simulink model "ESSController"  (R2020a)
settings: Solver=FixedStepAuto  StartTime=0.0  StopTime=10.0  FixedStep=1  RelTol=1e-3
libraries: ESSLibrary x19, simulink x1
settings Model: DataDictionary=ESSControllerData.sldd  EnableAccessToBaseWorkspace=off  Creator=soumyakantapanda  LastModifiedBy=soumyakantapanda

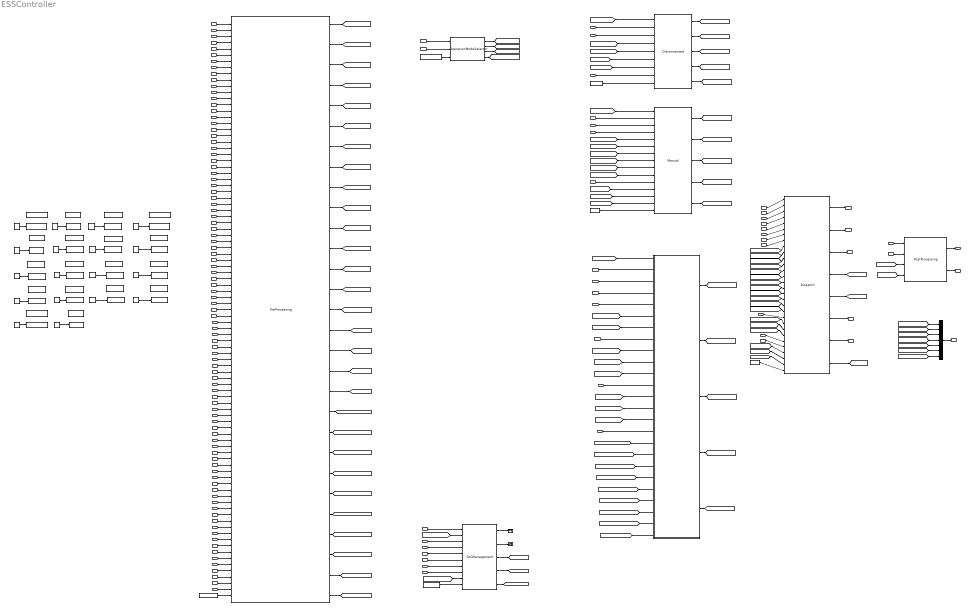
== system ESSController ==
  note: Dispatch and PostProcessing
  note: Auto Mode
  note: Manual Mode
  note: Disconnected Mode
  note: State of Charge Management Block
  note: Operation Mode Selection
  note: Pre-Processing
  note: LogicBlockIDGenerator
  EnablePreProcessing : Inport
  ActivePowerSet : Inport  Port=2
  ReactivePowerSet : Inport  Port=3
  ActivePowerMeasECP : Inport  Port=4
  ReactivePowerMeasECP : Inport  Port=5
  ActivePowerMeasCtrlPoint : Inport  Port=6
  ReactivePowerMeasCtrlPoint : Inport  Port=7
  FreqMeas : Inport  Port=8
  VoltMeasECPL1 : Inport  Port=9
  VoltMeasECPL2 : Inport  Port=10
  VoltMeasECPL3 : Inport  Port=11
  MaxDischargingPower : Inport  Port=12
  MaxChargingPower : Inport  Port=13
  ECPAppPow : Inport  Port=14
  RefFreq : Inport  Port=15
  RefVolt : Inport  Port=16
  TimeStep : Inport  Port=17
  BreakerCmdTime : Inport  Port=18
  OpenTimeOut : Inport  Port=19
  CloseTimeOut : Inport  Port=20
  ActivePowerRampUpRate : Inport  Port=21
  ActivePowerRampDownRate : Inport  Port=22
  ReactivePowerRampUpRate : Inport  Port=23
  ReactivePowerRampDownRate : Inport  Port=24
  VoltCloseThreshold : Inport  Port=25
  FreqCloseThreshold : Inport  Port=26
  ActivePowerOpenThreshold : Inport  Port=27
  ReactivePowerOpenThreshold : Inport  Port=28
  PQCapabilityCurveP1 : Inport  Port=29
  PQCapabilityCurveQ1 : Inport  Port=30
  PQCapabilityCurveP2 : Inport  Port=31
  PQCapabilityCurveQ2 : Inport  Port=32
  PQCapabilityCurveP3 : Inport  Port=33
  PQCapabilityCurveQ3 : Inport  Port=34
  PQCapabilityCurveP4 : Inport  Port=35
  PQCapabilityCurveQ4 : Inport  Port=36
  PQCapabilityCurveP5 : Inport  Port=37
  PQCapabilityCurveQ5 : Inport  Port=38
  PQCapabilityCurveP6 : Inport  Port=39
  PQCapabilityCurveQ6 : Inport  Port=40
  PQCapabilityCurveP7 : Inport  Port=41
  PQCapabilityCurveQ7 : Inport  Port=42
  PQCapabilityCurveP8 : Inport  Port=43
  PQCapabilityCurveQ8 : Inport  Port=44
  SoCTarget : Inport  Port=45
  MaxChOrDischDuration : Inport  Port=46
  BattCapacity : Inport  Port=47
  MaxImportPower : Inport  Port=48
  MaxExportPower : Inport  Port=49
  ActivePowerResponseReductionRatio : Inport  Port=50
  ActivePowerSmoothingLowDeadBand : Inport  Port=51
  ActivePowerSmoothingHighDeadBand : Inport  Port=52
  ActivePowerSmoothingGradient : Inport  Port=53
  ActivePowerSmoothingMovingAverageWindow : Inport  Port=54
  VoltWattHiStartVoltage : Inport  Port=55
  VoltWattHiStopVoltage : Inport  Port=56
  VoltWattHiVoltDischargeGradient : Inport  Port=57
  VoltWattHiVoltChargeGradient : Inport  Port=58
  VoltWattLoStartVoltage : Inport  Port=59
  VoltWattLoStopVoltage : Inport  Port=60
  VoltWattLoVoltDischargeGradient : Inport  Port=61
  VoltWattLoVoltChargeGradient : Inport  Port=62
  VoltWattStartDelay : Inport  Port=63
  VoltWattStopDelay : Inport  Port=64
  FreqWattHiStartFreq : Inport  Port=65
  FreqWattHiStopFreq : Inport  Port=66
  FreqWattHiFreqDischargeGradient : Inport  Port=67
  FreqWattHiFreqChargeGradient : Inport  Port=68
  FreqWattLoStartFreq : Inport  Port=69
  FreqWattLoStopFreq : Inport  Port=70
  FreqWattLoFreqDischargeGradient : Inport  Port=71
  FreqWattLoFreqChargeGradient : Inport  Port=72
  FreqWattStartDelay : Inport  Port=73
  FreqWattStopDelay : Inport  Port=74
  DynamicVoltWattLowDeadBand : Inport  Port=75
  DynamicVoltWattHighDeadBand : Inport  Port=76
  DynamicVoltWattGradient : Inport  Port=77
  DynamicVoltWattMovingAverageWindow : Inport  Port=78
  VoltVarHighStartingVoltage : Inport  Port=79
  VoltVarHighStoppingVoltage : Inport  Port=80
  VoltVarHighVoltageGradient : Inport  Port=81
  VoltVarLowStartingVoltage : Inport  Port=82
  VoltVarLowStoppingVoltage : Inport  Port=83
  VoltVarLowVoltageGradient : Inport  Port=84
  VoltVarOffsetReactivePower : Inport  Port=85
  WattVarHighStartingWattage : Inport  Port=86
  WattVarHighStoppingWattage : Inport  Port=87
  WattVarHighWattageGradient : Inport  Port=88
  WattVarLowStartingWattage : Inport  Port=89
  WattVarLowStoppingWattage : Inport  Port=90
  WattVarLowWattgeGradient : Inport  Port=91
  WattVarOffsetReactivePower : Inport  Port=92
  EnableOperationModeSelector : Inport  Port=93
  OperationMode : Inport  Port=94
  EnableSoCManagement : Inport  Port=95
  SoCMeas : Inport  Port=96
  SoCMin : Inport  Port=97
  SoCMax : Inport  Port=98
  CommQual : Inport  Port=99
  CBStatus : Inport  Port=100
  ResetDisconnected : Inport  Port=101
  OpenCmdIn : Inport  Port=102
  CloseCmdIn : Inport  Port=103
  ActivePowerControlMode : Inport  Port=104
  ReactivePowerControlMode : Inport  Port=105
  PowerFactorSet : Inport  Port=106
  ActivePowerLimitChargeOrDischarge : Inport  Port=107
  EnableDispatch : Inport  Port=108
  EnableRampLimiter : Inport  Port=109
  EnablePQCapabilityCurve : Inport  Port=110
  PQPriority : Inport  Port=111
  EnablePFLimit : Inport  Port=112
  PFOperMax : Inport  Port=113
  PFOperMin : Inport  Port=114
  EnablePostProcessing : Inport  Port=115
  ActivePowerControlMode1 : InportShadow  Port=104
  Auto : Subsystem
  BattCapacity1 : InportShadow  Port=47
  CBStatus1 : InportShadow  Port=100
  CBStatus2 : InportShadow  Port=100
  CommQual1 : InportShadow  Port=99
  CommQual2 : InportShadow  Port=99
  CommQual3 : InportShadow  Port=99
  Constant2 : Constant  OutDataTypeStr=int32  SampleTime=-1
  Constant3 : Constant  Value=2  OutDataTypeStr=int32  SampleTime=-1
  Constant37 : Constant  Value=7  OutDataTypeStr=int32  SampleTime=-1
  Constant38 : Constant  Value=8  OutDataTypeStr=int32  SampleTime=-1
  Constant4 : Constant  Value=3  OutDataTypeStr=int32  SampleTime=-1
  Constant40 : Constant  Value=9  OutDataTypeStr=int32  SampleTime=-1
  Constant41 : Constant  Value=10  OutDataTypeStr=int32  SampleTime=-1
  Constant42 : Constant  Value=11  OutDataTypeStr=int32  SampleTime=-1
  Constant43 : Constant  Value=12  OutDataTypeStr=int32  SampleTime=-1
  Constant44 : Constant  Value=13  OutDataTypeStr=int32  SampleTime=-1
  Constant45 : Constant  Value=14  OutDataTypeStr=int32  SampleTime=-1
  Constant46 : Constant  Value=15  OutDataTypeStr=int32  SampleTime=-1
  Constant47 : Constant  Value=16  OutDataTypeStr=int32  SampleTime=-1
  Constant48 : Constant  Value=17  OutDataTypeStr=int32  SampleTime=-1
  Constant5 : Constant  Value=4  OutDataTypeStr=int32  SampleTime=-1
  Constant6 : Constant  Value=5  OutDataTypeStr=int32  SampleTime=-1
  Constant8 : Constant  Value=18  OutDataTypeStr=int32  SampleTime=-1
  Constant9 : Constant  Value=8  OutDataTypeStr=int64  SampleTime=-1
  Data Store Memory2 : DataStoreMemory  DataStoreName=OperationModeSelector  ShowAdditionalParam=off
  Data Store Memory3 : DataStoreMemory  DataStoreName=SoCComparator  ShowAdditionalParam=off
  Data Store Memory35 : DataStoreMemory  DataStoreName=ChargeDischargeStorageMode  ShowAdditionalParam=off
  Data Store Memory36 : DataStoreMemory  DataStoreName=CoordinatedChDisMode  ShowAdditionalParam=off
  Data Store Memory38 : DataStoreMemory  DataStoreName=ActivePowResponseMode  ShowAdditionalParam=off
  Data Store Memory39 : DataStoreMemory  DataStoreName=ActivePowSmoothingMode  ShowAdditionalParam=off
  Data Store Memory4 : DataStoreMemory  DataStoreName=PreProcessingBlock  ShowAdditionalParam=off
  Data Store Memory40 : DataStoreMemory  DataStoreName=VoltWattMode  ShowAdditionalParam=off
  Data Store Memory41 : DataStoreMemory  DataStoreName=FreqWattMode  ShowAdditionalParam=off
  Data Store Memory42 : DataStoreMemory  DataStoreName=DynamicVoltWattMode  ShowAdditionalParam=off
  Data Store Memory43 : DataStoreMemory  DataStoreName=ConstVARMode  ShowAdditionalParam=off
  Data Store Memory44 : DataStoreMemory  DataStoreName=FixedPFMode  ShowAdditionalParam=off
  Data Store Memory45 : DataStoreMemory  DataStoreName=VoltVARMode  ShowAdditionalParam=off
  Data Store Memory46 : DataStoreMemory  DataStoreName=WattVARMode  ShowAdditionalParam=off
  Data Store Memory5 : DataStoreMemory  DataStoreName=Disconnected  ShowAdditionalParam=off
  Data Store Memory6 : DataStoreMemory  DataStoreName=Manual  ShowAdditionalParam=off
  Data Store Memory8 : DataStoreMemory  DataStoreName=Dispatch  ShowAdditionalParam=off
  Data Store Memory9 : DataStoreMemory  DataStoreName=PostProcessing  ShowAdditionalParam=off
  Data Store Read : DataStoreRead  DataStoreName=PreProcessingBlock
  Data Store Read1 : DataStoreRead  DataStoreName=OperationModeSelector
  Data Store Read2 : DataStoreRead  DataStoreName=SoCComparator
  Data Store Read3 : DataStoreRead  DataStoreName=Disconnected
  Data Store Read4 : DataStoreRead  DataStoreName=Manual
  Data Store Read5 : DataStoreRead  DataStoreName=Dispatch
  Data Store Write2 : DataStoreWrite  DataStoreName=SoCComparator
  Data Store Write3 : DataStoreWrite  DataStoreName=OperationModeSelector
  Data Store Write35 : DataStoreWrite  DataStoreName=ChargeDischargeStorageMode
  Data Store Write36 : DataStoreWrite  DataStoreName=CoordinatedChDisMode
  Data Store Write38 : DataStoreWrite  DataStoreName=ActivePowResponseMode
  Data Store Write39 : DataStoreWrite  DataStoreName=ActivePowSmoothingMode
  Data Store Write4 : DataStoreWrite  DataStoreName=PreProcessingBlock
  Data Store Write40 : DataStoreWrite  DataStoreName=VoltWattMode
  Data Store Write41 : DataStoreWrite  DataStoreName=FreqWattMode
  Data Store Write42 : DataStoreWrite  DataStoreName=DynamicVoltWattMode
  Data Store Write43 : DataStoreWrite  DataStoreName=ConstVARMode
  Data Store Write44 : DataStoreWrite  DataStoreName=FixedPFMode
  Data Store Write45 : DataStoreWrite  DataStoreName=VoltVARMode
  Data Store Write46 : DataStoreWrite  DataStoreName=WattVARMode
  Data Store Write5 : DataStoreWrite  DataStoreName=Manual
  Data Store Write6 : DataStoreWrite  DataStoreName=Disconnected
  Data Store Write8 : DataStoreWrite  DataStoreName=PostProcessing
  Data Store Write9 : DataStoreWrite  DataStoreName=Dispatch
  Disconnected : ESSLibrary/Disconnected  SystemSampleTime=-1  Latency=0  AutoFrameSizeCalculation=off
  Dispatch : ESSLibrary/Dispatch  SystemSampleTime=-1  Latency=0  AutoFrameSizeCalculation=off
  ECPAppPow1 : InportShadow  Port=14
  ECPAppPow2 : InportShadow  Port=14
  Manual : ESSLibrary/Manual  SystemSampleTime=-1  Latency=0  AutoFrameSizeCalculation=off
  Mux : Mux  Inputs=7
  OperationMode1 : InportShadow  Port=94
  OperationModeSelector : ESSLibrary/OperationModeSelector  SystemSampleTime=-1  Latency=0  AutoFrameSizeCalculation=off
  PostProcessing : ESSLibrary/PostProcessing  SystemSampleTime=-1  Latency=0  AutoFrameSizeCalculation=off
  PreProcessing : ESSLibrary/PreProcessing  SystemSampleTime=-1  Latency=0  AutoFrameSizeCalculation=off
  ReactivePowerControlMode1 : InportShadow  Port=105
  SoCManagement : ESSLibrary/SoCManagement  SystemSampleTime=-1  Latency=0  AutoFrameSizeCalculation=off
  SoCMeas1 : InportShadow  Port=96
  Terminator : Terminator
  Terminator1 : Terminator
  TimeStep1 : InportShadow  Port=17
  OperationModeOut : Outport  SignalName=OperationModeOut
  ActivePowerModeOut : Outport  Port=2  SignalName=ActivePowerModeOut
  ReactivePowerModeOut : Outport  Port=3  SignalName=ReactivePowerModeOut
  OpenCmdOut : Outport  Port=4  SignalName=OpenCmdOut
  CloseCmdOut : Outport  Port=5  SignalName=CloseCmdOut
  ActivePowerOut : Outport  Port=6  SignalName=ActivePowerOut
  ReactivePowerOut : Outport  Port=7  SignalName=ReactivePowerOut
  ErrorCode : Outport  Port=8  SignalName=ErrorCode
  wires:
  Constant38/1 -> Data Store Write36/1
  Constant8/1 -> Data Store Write9/1
  Constant43/1 -> Data Store Write41/1
  Constant42/1 -> Data Store Write40/1
  Constant48/1 -> Data Store Write46/1
  Constant47/1 -> Data Store Write45/1
  Constant46/1 -> Data Store Write44/1
  Constant45/1 -> Data Store Write43/1
  Constant40/1 -> Data Store Write38/1
  Constant44/1 -> Data Store Write42/1
  Constant37/1 -> Data Store Write35/1
  Constant2/1 -> Data Store Write3/1
  Constant6/1 -> Data Store Write5/1
  Constant3/1 -> Data Store Write2/1
  Constant5/1 -> Data Store Write6/1
  Constant9/1 -> Data Store Write8/1
  Constant41/1 -> Data Store Write39/1
  Constant4/1 -> Data Store Write4/1
  EnablePreProcessing/1 -> PreProcessing/1
  ActivePowerSet/1 -> PreProcessing/2
  ReactivePowerSet/1 -> PreProcessing/3
  ActivePowerMeasECP/1 -> PreProcessing/4
  ReactivePowerMeasECP/1 -> PreProcessing/5
  ActivePowerMeasCtrlPoint/1 -> PreProcessing/6
  ReactivePowerMeasCtrlPoint/1 -> PreProcessing/7
  FreqMeas/1 -> PreProcessing/8
  VoltMeasECPL1/1 -> PreProcessing/9
  VoltMeasECPL2/1 -> PreProcessing/10
  VoltMeasECPL3/1 -> PreProcessing/11
  MaxDischargingPower/1 -> PreProcessing/12
  ReactivePowerRampDownRate/1 -> PreProcessing/24
  ReactivePowerRampUpRate/1 -> PreProcessing/23
  ActivePowerRampDownRate/1 -> PreProcessing/22
  ActivePowerRampUpRate/1 -> PreProcessing/21
  CloseTimeOut/1 -> PreProcessing/20
  OpenTimeOut/1 -> PreProcessing/19
  BreakerCmdTime/1 -> PreProcessing/18
  TimeStep/1 -> PreProcessing/17
  RefVolt/1 -> PreProcessing/16
  RefFreq/1 -> PreProcessing/15
  ECPAppPow/1 -> PreProcessing/14
  MaxChargingPower/1 -> PreProcessing/13
  PQCapabilityCurveP5/1 -> PreProcessing/37
  PQCapabilityCurveQ5/1 -> PreProcessing/38
  PQCapabilityCurveP6/1 -> PreProcessing/39
  PQCapabilityCurveQ6/1 -> PreProcessing/40
  PQCapabilityCurveP7/1 -> PreProcessing/41
  PQCapabilityCurveQ7/1 -> PreProcessing/42
  PQCapabilityCurveP8/1 -> PreProcessing/43
  PQCapabilityCurveQ8/1 -> PreProcessing/44
  SoCTarget/1 -> PreProcessing/45
  MaxChOrDischDuration/1 -> PreProcessing/46
  BattCapacity/1 -> PreProcessing/47
  MaxImportPower/1 -> PreProcessing/48
  PQCapabilityCurveQ4/1 -> PreProcessing/36
  PQCapabilityCurveP4/1 -> PreProcessing/35
  PQCapabilityCurveQ3/1 -> PreProcessing/34
  PQCapabilityCurveP3/1 -> PreProcessing/33
  PQCapabilityCurveQ2/1 -> PreProcessing/32
  PQCapabilityCurveP2/1 -> PreProcessing/31
  PQCapabilityCurveQ1/1 -> PreProcessing/30
  PQCapabilityCurveP1/1 -> PreProcessing/29
  ReactivePowerOpenThreshold/1 -> PreProcessing/28
  ActivePowerOpenThreshold/1 -> PreProcessing/27
  FreqCloseThreshold/1 -> PreProcessing/26
  VoltCloseThreshold/1 -> PreProcessing/25
  FreqWattStartDelay/1 -> PreProcessing/73
  FreqWattStopDelay/1 -> PreProcessing/74
  DynamicVoltWattLowDeadBand/1 -> PreProcessing/75
  DynamicVoltWattHighDeadBand/1 -> PreProcessing/76
  DynamicVoltWattGradient/1 -> PreProcessing/77
  DynamicVoltWattMovingAverageWindow/1 -> PreProcessing/78
  VoltVarHighStartingVoltage/1 -> PreProcessing/79
  VoltVarHighStoppingVoltage/1 -> PreProcessing/80
  VoltVarHighVoltageGradient/1 -> PreProcessing/81
  VoltVarLowStartingVoltage/1 -> PreProcessing/82
  VoltVarLowStoppingVoltage/1 -> PreProcessing/83
  VoltVarLowVoltageGradient/1 -> PreProcessing/84
  Data Store Read/1 -> PreProcessing/93
  WattVarOffsetReactivePower/1 -> PreProcessing/92
  WattVarLowWattgeGradient/1 -> PreProcessing/91
  WattVarLowStoppingWattage/1 -> PreProcessing/90
  WattVarLowStartingWattage/1 -> PreProcessing/89
  WattVarHighWattageGradient/1 -> PreProcessing/88
  WattVarHighStoppingWattage/1 -> PreProcessing/87
  WattVarHighStartingWattage/1 -> PreProcessing/86
  VoltVarOffsetReactivePower/1 -> PreProcessing/85
  VoltWattLoVoltDischargeGradient/1 -> PreProcessing/61
  VoltWattLoVoltChargeGradient/1 -> PreProcessing/62
  VoltWattStartDelay/1 -> PreProcessing/63
  VoltWattStopDelay/1 -> PreProcessing/64
  FreqWattHiStartFreq/1 -> PreProcessing/65
  FreqWattHiStopFreq/1 -> PreProcessing/66
  FreqWattHiFreqDischargeGradient/1 -> PreProcessing/67
  FreqWattHiFreqChargeGradient/1 -> PreProcessing/68
  FreqWattLoStartFreq/1 -> PreProcessing/69
  FreqWattLoStopFreq/1 -> PreProcessing/70
  FreqWattLoFreqDischargeGradient/1 -> PreProcessing/71
  FreqWattLoFreqChargeGradient/1 -> PreProcessing/72
  VoltWattLoStopVoltage/1 -> PreProcessing/60
  VoltWattLoStartVoltage/1 -> PreProcessing/59
  VoltWattHiVoltChargeGradient/1 -> PreProcessing/58
  VoltWattHiVoltDischargeGradient/1 -> PreProcessing/57
  VoltWattHiStopVoltage/1 -> PreProcessing/56
  VoltWattHiStartVoltage/1 -> PreProcessing/55
  ActivePowerSmoothingMovingAverageWindow/1 -> PreProcessing/54
  ActivePowerSmoothingGradient/1 -> PreProcessing/53
  ActivePowerSmoothingHighDeadBand/1 -> PreProcessing/52
  ActivePowerSmoothingLowDeadBand/1 -> PreProcessing/51
  ActivePowerResponseReductionRatio/1 -> PreProcessing/50
  MaxExportPower/1 -> PreProcessing/49
  PreProcessing/1 -> [ActivePowerSetPU]
  PreProcessing/2 -> [ReactivePowerSetPU]
  PreProcessing/3 -> [ActivePowerMeasPU]
  PreProcessing/4 -> [ReactivePowerMeasPU]
  PreProcessing/5 -> [ActivePowerMeasCtrlPointPU]
  PreProcessing/6 -> [ReactivePowerMeasCtrlPointPU]
  PreProcessing/7 -> [FreqMeasPU]
  PreProcessing/8 -> [VoltMeasPU]
  PreProcessing/9 -> [MaxDischargingPowerPU]
  PreProcessing/10 -> [MaxChargingPowerPU]
  PreProcessing/11 -> [FreqWithinLimits]
  PreProcessing/12 -> [VoltWithinLimits]
  PreProcessing/13 -> [ZeroActivePowerFlow]
  PreProcessing/14 -> [ZeroReactivePowerFlow]
  PreProcessing/15 -> [ActiveReactiveRampUpDownData]
  PreProcessing/16 -> [PQCapabilityCurvePU]
  PreProcessing/17 -> [BreakerCmdTimeSteps]
  PreProcessing/18 -> [OpenTimeOutTimeSteps]
  PreProcessing/19 -> [CloseTimeOutTimeSteps]
  PreProcessing/20 -> [ActivePowerLimitOperatingParametersPU]
  PreProcessing/21 -> [CrdChargeDischargeOperatingParametersPU]
  PreProcessing/22 -> [ActivePowerResponseOperatingParametersPU]
  PreProcessing/23 -> [ActivePowerSmoothingOperatingParametersPU]
  PreProcessing/24 -> [VoltWattOperatingParametersPU]
  PreProcessing/25 -> [FreqWattOperatingParametersPU]
  PreProcessing/26 -> [DynamicVoltWattOperatingParametersPU]
  PreProcessing/27 -> [VoltVAROperatingParametersPU]
  PreProcessing/28 -> [WattVAROperatingParametersPU]
  PreProcessing/29 -> [PreProcessingErrorCode]
  EnableOperationModeSelector/1 -> OperationModeSelector/1
  OperationMode/1 -> OperationModeSelector/2
  Data Store Read1/1 -> OperationModeSelector/3
  OperationModeSelector/3 -> [EnableAutoMode]
  OperationModeSelector/1 -> [EnableDisconnectedMode]
  OperationModeSelector/4 -> [OperationModeSelectorErrorCode]
  OperationModeSelector/2 -> [EnableManualMode]
  EnableSoCManagement/1 -> SoCManagement/1
  [ActivePowerMeasPU] -> SoCManagement/2
  SoCMeas/1 -> SoCManagement/3
  SoCMin/1 -> SoCManagement/4
  SoCMax/1 -> SoCManagement/5
  BattCapacity1/1 -> SoCManagement/6
  ECPAppPow1/1 -> SoCManagement/7
  TimeStep1/1 -> SoCManagement/8
  [ActiveReactiveRampUpDownData] -> SoCManagement/9
  Data Store Read2/1 -> SoCManagement/10
  SoCManagement/1 -> Terminator/1
  SoCManagement/2 -> Terminator1/1
  SoCManagement/3 -> [ChargeEnable]
  SoCManagement/4 -> [DischargeEnable]
  SoCManagement/5 -> [SoCManagementErrorCode]
  [EnableDisconnectedMode] -> Disconnected/1
  CommQual/1 -> Disconnected/2
  CBStatus/1 -> Disconnected/3
  [ZeroActivePowerFlow] -> Disconnected/4
  [ZeroReactivePowerFlow] -> Disconnected/5
  [BreakerCmdTimeSteps] -> Disconnected/6
  [OpenTimeOutTimeSteps] -> Disconnected/7
  ResetDisconnected/1 -> Disconnected/8
  Data Store Read3/1 -> Disconnected/9
  Disconnected/1 -> [ActivePowerOutDisconnected]
  Disconnected/2 -> [ReactivePowerOutDisconnected]
  Disconnected/3 -> [OpenCmdDisconnected]
  Disconnected/4 -> [CloseCmdDisconnected]
  Disconnected/5 -> [DisconnectedErrorCode]
  [EnableManualMode] -> Manual/1
  CommQual1/1 -> Manual/2
  CBStatus1/1 -> Manual/11
  OpenCmdIn/1 -> Manual/3
  CloseCmdIn/1 -> Manual/4
  [FreqWithinLimits] -> Manual/5
  [VoltWithinLimits] -> Manual/6
  [ZeroActivePowerFlow] -> Manual/9
  [ZeroReactivePowerFlow] -> Manual/10
  [ActivePowerSetPU] -> Manual/7
  [ReactivePowerSetPU] -> Manual/8
  [OpenTimeOutTimeSteps] -> Manual/13
  [BreakerCmdTimeSteps] -> Manual/12
  [CloseTimeOutTimeSteps] -> Manual/14
  Data Store Read4/1 -> Manual/15
  Manual/1 -> [ActivePowerOutManual]
  Manual/2 -> [ReactivePowerOutManual]
  Manual/3 -> [OpenCmdManual]
  Manual/4 -> [CloseCmdManual]
  Manual/5 -> [ManualErrorCode]
  [EnableAutoMode] -> Auto/1(Enable)
  CommQual2/1 -> Auto/2(CommQual)
  CBStatus2/1 -> Auto/3(CBStatus)
  ActivePowerControlMode/1 -> Auto/4(ActivePowerControlMode)
  ReactivePowerControlMode/1 -> Auto/5(ReactivePowerControlMode)
  [ActivePowerSetPU] -> Auto/6(ActivePowerSetPU)
  [ReactivePowerSetPU] -> Auto/7(ReactivePowerSetPU)
  [ActivePowerMeasPU] -> Auto/9(ActivePowerMeasPU)
  [ActivePowerMeasCtrlPointPU] -> Auto/13(ActivePowerMeasCtrlPointPU)
  [VoltMeasPU] -> Auto/10(VoltMeasPU)
  [FreqMeasPU] -> Auto/11(FreqMeasPU)
  [MaxDischargingPowerPU] -> Auto/14(MaxDischargingPowerPU)
  [MaxChargingPowerPU] -> Auto/15(MaxChargingPowerPU)
  SoCMeas1/1 -> Auto/12(SoCMeas)
  PowerFactorSet/1 -> Auto/8(PowerFactorSet)
  ActivePowerLimitChargeOrDischarge/1 -> Auto/16(ActivePowerLimitChargeOrDischarge)
  [ActivePowerLimitOperatingParametersPU] -> Auto/17(ActivePowerLimitOperatingParametersPU)
  [CrdChargeDischargeOperatingParametersPU] -> Auto/18(CrdChargeDischargeOperatingParametersPU)
  [ActivePowerResponseOperatingParametersPU] -> Auto/19(ActivePowerResponseOperatingParametersPU)
  [VoltWattOperatingParametersPU] -> Auto/20(VoltWattOperatingParametersPU)
  [FreqWattOperatingParametersPU] -> Auto/21(FreqWattOperatingParametersPU)
  [ActivePowerSmoothingOperatingParametersPU] -> Auto/22(ActivePowerSmoothingOperatingParametersPU)
  [DynamicVoltWattOperatingParametersPU] -> Auto/23(DynamicVoltWattOperatingParametersPU)
  [VoltVAROperatingParametersPU] -> Auto/24(VoltVAROperatingParametersPU)
  [WattVAROperatingParametersPU] -> Auto/25(WattVAROperatingParametersPU)
  Auto/1(ActivePowerOut) -> [ActivePowerOutAuto]
  Auto/2(ReactivePowerOut) -> [ReactivePowerOutAuto]
  Auto/3(OpenCmd) -> [OpenCmdAuto]
  Auto/4(CloseCmd) -> [CloseCmdAuto]
  Auto/5(ErrorCode) -> [AutoErrorCode]
  EnableDispatch/1 -> Dispatch/1
  OperationMode1/1 -> Dispatch/2
  ActivePowerControlMode1/1 -> Dispatch/3
  ReactivePowerControlMode1/1 -> Dispatch/4
  EnableRampLimiter/1 -> Dispatch/5
  EnablePQCapabilityCurve/1 -> Dispatch/6
  EnablePFLimit/1 -> Dispatch/7
  [ActivePowerOutDisconnected] -> Dispatch/9
  [ActivePowerOutManual] -> Dispatch/10
  [ReactivePowerOutAuto] -> Dispatch/14
  [OpenCmdDisconnected] -> Dispatch/15
  [ActivePowerOutAuto] -> Dispatch/11
  [OpenCmdManual] -> Dispatch/16
  [CloseCmdAuto] -> Dispatch/20
  [ReactivePowerOutManual] -> Dispatch/13
  [OpenCmdAuto] -> Dispatch/17
  [CloseCmdDisconnected] -> Dispatch/18
  [CloseCmdManual] -> Dispatch/19
  [ActiveReactiveRampUpDownData] -> Dispatch/22
  [ReactivePowerOutDisconnected] -> Dispatch/12
  [ActivePowerMeasPU] -> Dispatch/23
  [ReactivePowerMeasPU] -> Dispatch/24
  PQPriority/1 -> Dispatch/8
  CommQual3/1 -> Dispatch/21
  [PQCapabilityCurvePU] -> Dispatch/27
  PFOperMax/1 -> Dispatch/25
  PFOperMin/1 -> Dispatch/26
  [ChargeEnable] -> Dispatch/28
  [DischargeEnable] -> Dispatch/29
  Data Store Read5/1 -> Dispatch/30
  Dispatch/1 -> OperationModeOut/1
  Dispatch/2 -> ActivePowerModeOut/1
  Dispatch/3 -> ReactivePowerModeOut/1
  Dispatch/4 -> [ActivePowerOutPU]
  Dispatch/5 -> [ReactivePowerOutPU]
  Dispatch/6 -> OpenCmdOut/1
  Dispatch/7 -> CloseCmdOut/1
  Dispatch/8 -> [DispatchErrorCode]
  [ActivePowerOutPU] -> PostProcessing/3
  [ReactivePowerOutPU] -> PostProcessing/4
  ECPAppPow2/1 -> PostProcessing/2
  EnablePostProcessing/1 -> PostProcessing/1
  PostProcessing/1 -> ActivePowerOut/1
  PostProcessing/2 -> ReactivePowerOut/1
  Mux/1 -> ErrorCode/1
  [ManualErrorCode] -> Mux/5
  [AutoErrorCode] -> Mux/6
  [DispatchErrorCode] -> Mux/7
  [OperationModeSelectorErrorCode] -> Mux/1
  [SoCManagementErrorCode] -> Mux/2
  [PreProcessingErrorCode] -> Mux/3
  [DisconnectedErrorCode] -> Mux/4

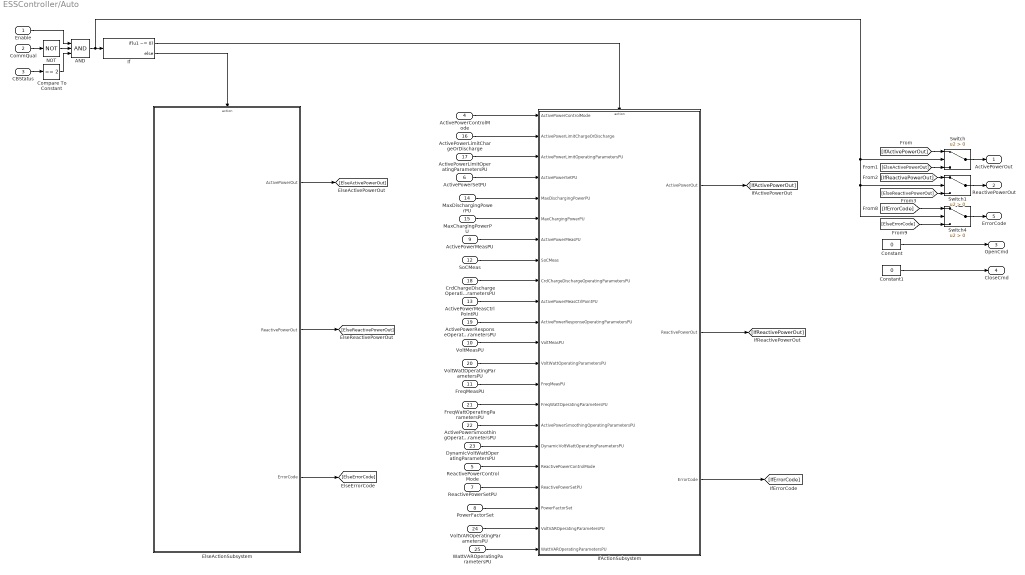
== system ESSController/Auto ==
  Enable : Inport
  CommQual : Inport  Port=2  OutDataTypeStr=boolean
  CBStatus : Inport  Port=3
  ActivePowerControlMode : Inport  Port=4
  ReactivePowerControlMode : Inport  Port=5
  ActivePowerSetPU : Inport  Port=6
  ReactivePowerSetPU : Inport  Port=7
  PowerFactorSet : Inport  Port=8
  ActivePowerMeasPU : Inport  Port=9
  VoltMeasPU : Inport  Port=10
  FreqMeasPU : Inport  Port=11
  SoCMeas : Inport  Port=12
  ActivePowerMeasCtrlPointPU : Inport  Port=13
  MaxDischargingPowerPU : Inport  Port=14
  MaxChargingPowerPU : Inport  Port=15
  ActivePowerLimitChargeOrDischarge : Inport  Port=16
  ActivePowerLimitOperatingParametersPU : Inport  Port=17  OutDataTypeStr=Bus: ActivePowerLimitOperatingParametersPU
  CrdChargeDischargeOperatingParametersPU : Inport  Port=18  OutDataTypeStr=Bus: CrdChargeDischargeOperatingParametersPU
  ActivePowerResponseOperatingParametersPU : Inport  Port=19  OutDataTypeStr=Bus: ActivePowerResponseOperatingParametersPU
  VoltWattOperatingParametersPU : Inport  Port=20  OutDataTypeStr=Bus: VoltWattOperatingParametersPU
  FreqWattOperatingParametersPU : Inport  Port=21  OutDataTypeStr=Bus: FreqWattOperatingParametersPU
  ActivePowerSmoothingOperatingParametersPU : Inport  Port=22  OutDataTypeStr=Bus: ActivePowerSmoothingOperatingParametersPU
  DynamicVoltWattOperatingParametersPU : Inport  Port=23  OutDataTypeStr=Bus: DynamicVoltWattOperatingParametersPU
  VoltVAROperatingParametersPU : Inport  Port=24  OutDataTypeStr=Bus: VoltVarOperatingParametersPU
  WattVAROperatingParametersPU : Inport  Port=25  OutDataTypeStr=Bus: WattVarOperatingParametersPU
  AND : Logic  Inputs=3  IconShape=distinctive  AllPortsSameDT=off  OutDataTypeStr=boolean
  Compare To Constant : simulink/Logic and Bit Operations/Compare To Constant  relop===  const=2  OutDataTypeStr=boolean
  Constant : Constant  Value=0  OutDataTypeStr=boolean  SampleTime=-1
  Constant1 : Constant  Value=0  OutDataTypeStr=boolean  SampleTime=-1
  ElseActionSubsystem : Subsystem  TreatAsAtomicUnit=on
  If : If  IfExpression=u1 ~= 0
  IfActionSubsystem : Subsystem  TreatAsAtomicUnit=on
  NOT : Logic  Operator=NOT  IconShape=distinctive  AllPortsSameDT=off  OutDataTypeStr=boolean
  Switch : Switch  Criteria=u2 > Threshold
  Switch1 : Switch  Criteria=u2 > Threshold
  Switch4 : Switch  Criteria=u2 > Threshold
  ActivePowerOut : Outport
  ReactivePowerOut : Outport  Port=2
  OpenCmd : Outport  Port=3
  CloseCmd : Outport  Port=4
  ErrorCode : Outport  Port=5  OutDataTypeStr=int64
  wires:
  If/2 -> ElseActionSubsystem/Action
  If/1 -> IfActionSubsystem/Action
  ActivePowerControlMode/1 -> IfActionSubsystem/1(ActivePowerControlMode)
  ReactivePowerControlMode/1 -> IfActionSubsystem/18(ReactivePowerControlMode)
  ActivePowerLimitChargeOrDischarge/1 -> IfActionSubsystem/2(ActivePowerLimitChargeOrDischarge)
  ActivePowerLimitOperatingParametersPU/1 -> IfActionSubsystem/3(ActivePowerLimitOperatingParametersPU)
  ActivePowerSetPU/1 -> IfActionSubsystem/4(ActivePowerSetPU)
  MaxDischargingPowerPU/1 -> IfActionSubsystem/5(MaxDischargingPowerPU)
  MaxChargingPowerPU/1 -> IfActionSubsystem/6(MaxChargingPowerPU)
  ActivePowerMeasPU/1 -> IfActionSubsystem/7(ActivePowerMeasPU)
  SoCMeas/1 -> IfActionSubsystem/8(SoCMeas)
  CrdChargeDischargeOperatingParametersPU/1 -> IfActionSubsystem/9(CrdChargeDischargeOperatingParametersPU)
  ActivePowerMeasCtrlPointPU/1 -> IfActionSubsystem/10(ActivePowerMeasCtrlPointPU)
  ActivePowerResponseOperatingParametersPU/1 -> IfActionSubsystem/11(ActivePowerResponseOperatingParametersPU)
  VoltMeasPU/1 -> IfActionSubsystem/12(VoltMeasPU)
  VoltWattOperatingParametersPU/1 -> IfActionSubsystem/13(VoltWattOperatingParametersPU)
  FreqMeasPU/1 -> IfActionSubsystem/14(FreqMeasPU)
  FreqWattOperatingParametersPU/1 -> IfActionSubsystem/15(FreqWattOperatingParametersPU)
  ActivePowerSmoothingOperatingParametersPU/1 -> IfActionSubsystem/16(ActivePowerSmoothingOperatingParametersPU)
  DynamicVoltWattOperatingParametersPU/1 -> IfActionSubsystem/17(DynamicVoltWattOperatingParametersPU)
  ReactivePowerSetPU/1 -> IfActionSubsystem/19(ReactivePowerSetPU)
  PowerFactorSet/1 -> IfActionSubsystem/20(PowerFactorSet)
  VoltVAROperatingParametersPU/1 -> IfActionSubsystem/21(VoltVAROperatingParametersPU)
  WattVAROperatingParametersPU/1 -> IfActionSubsystem/22(WattVAROperatingParametersPU)
  ElseActionSubsystem/1(ActivePowerOut) -> [ElseActivePowerOut]
  ElseActionSubsystem/2(ReactivePowerOut) -> [ElseReactivePowerOut]
  ElseActionSubsystem/3(ErrorCode) -> [ElseErrorCode]
  IfActionSubsystem/1(ActivePowerOut) -> [IfActivePowerOut]
  IfActionSubsystem/2(ReactivePowerOut) -> [IfReactivePowerOut]
  IfActionSubsystem/3(ErrorCode) -> [IfErrorCode]
  CommQual/1 -> NOT/1
  NOT/1 -> AND/2
  Enable/1 -> AND/1
  CBStatus/1 -> Compare To Constant/1
  Compare To Constant/1 -> AND/3
  [IfActivePowerOut] -> Switch/1
  [ElseErrorCode] -> Switch4/3
  [ElseActivePowerOut] -> Switch/3
  [ElseReactivePowerOut] -> Switch1/3
  AND/1 -> Switch/2, Switch1/2, Switch4/2, If/1
  [IfReactivePowerOut] -> Switch1/1
  Switch4/1 -> ErrorCode/1
  Switch/1 -> ActivePowerOut/1
  Switch1/1 -> ReactivePowerOut/1
  [IfErrorCode] -> Switch4/1
  Constant/1 -> OpenCmd/1
  Constant1/1 -> CloseCmd/1

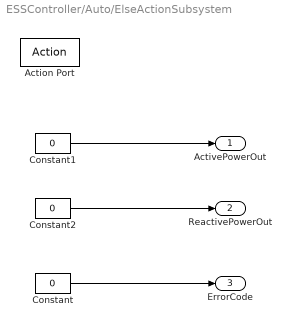
== system ESSController/Auto/ElseActionSubsystem ==
  Action Port : ActionPort
  Constant : Constant  Value=0  OutDataTypeStr=int32  SampleTime=-1
  Constant1 : Constant  Value=0  OutDataTypeStr=double  SampleTime=-1
  Constant2 : Constant  Value=0  OutDataTypeStr=double  SampleTime=-1
  ActivePowerOut : Outport
  ReactivePowerOut : Outport  Port=2
  ErrorCode : Outport  Port=3
  wires:
  Constant/1 -> ErrorCode/1
  Constant1/1 -> ActivePowerOut/1
  Constant2/1 -> ReactivePowerOut/1

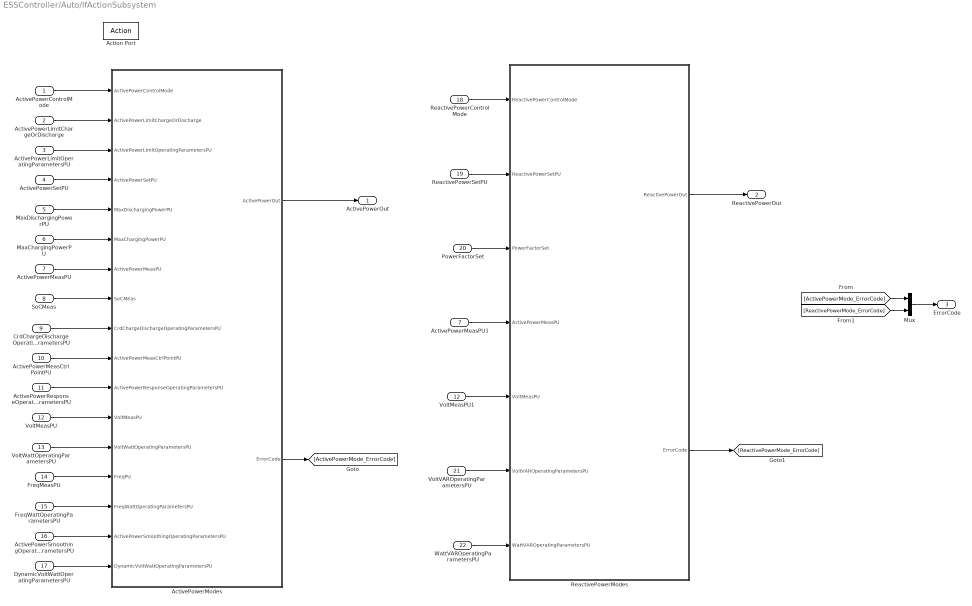
== system ESSController/Auto/IfActionSubsystem ==
  ActivePowerControlMode : Inport
  ActivePowerLimitChargeOrDischarge : Inport  Port=2
  ActivePowerLimitOperatingParametersPU : Inport  Port=3  OutDataTypeStr=Bus: ActivePowerLimitOperatingParametersPU
  ActivePowerSetPU : Inport  Port=4
  MaxDischargingPowerPU : Inport  Port=5
  MaxChargingPowerPU : Inport  Port=6
  ActivePowerMeasPU : Inport  Port=7
  SoCMeas : Inport  Port=8
  CrdChargeDischargeOperatingParametersPU : Inport  Port=9  OutDataTypeStr=Bus: CrdChargeDischargeOperatingParametersPU
  ActivePowerMeasCtrlPointPU : Inport  Port=10
  ActivePowerResponseOperatingParametersPU : Inport  Port=11  OutDataTypeStr=Bus: ActivePowerResponseOperatingParametersPU
  VoltMeasPU : Inport  Port=12
  VoltWattOperatingParametersPU : Inport  Port=13  OutDataTypeStr=Bus: VoltWattOperatingParametersPU
  FreqMeasPU : Inport  Port=14
  FreqWattOperatingParametersPU : Inport  Port=15  OutDataTypeStr=Bus: FreqWattOperatingParametersPU
  ActivePowerSmoothingOperatingParametersPU : Inport  Port=16  OutDataTypeStr=Bus: ActivePowerSmoothingOperatingParametersPU
  DynamicVoltWattOperatingParametersPU : Inport  Port=17  OutDataTypeStr=Bus: DynamicVoltWattOperatingParametersPU
  ReactivePowerControlMode : Inport  Port=18
  ReactivePowerSetPU : Inport  Port=19
  PowerFactorSet : Inport  Port=20
  VoltVAROperatingParametersPU : Inport  Port=21  OutDataTypeStr=Bus: VoltVarOperatingParametersPU
  WattVAROperatingParametersPU : Inport  Port=22  OutDataTypeStr=Bus: WattVarOperatingParametersPU
  Action Port : ActionPort
  ActivePowerMeasPU1 : InportShadow  Port=7
  ActivePowerModes : Subsystem
  Mux : Mux  Inputs=2
  ReactivePowerModes : Subsystem
  VoltMeasPU1 : InportShadow  Port=12
  ActivePowerOut : Outport
  ReactivePowerOut : Outport  Port=2
  ErrorCode : Outport  Port=3
  wires:
  ActivePowerModes/1(ActivePowerOut) -> ActivePowerOut/1
  ReactivePowerModes/1(ReactivePowerOut) -> ReactivePowerOut/1
  ActivePowerModes/2(ErrorCode) -> [ActivePowerMode_ErrorCode]
  ReactivePowerModes/2(ErrorCode) -> [ReactivePowerMode_ErrorCode]
  Mux/1 -> ErrorCode/1
  [ActivePowerMode_ErrorCode] -> Mux/1
  [ReactivePowerMode_ErrorCode] -> Mux/2
  ActivePowerControlMode/1 -> ActivePowerModes/1(ActivePowerControlMode)
  ActivePowerLimitChargeOrDischarge/1 -> ActivePowerModes/2(ActivePowerLimitChargeOrDischarge)
  ActivePowerLimitOperatingParametersPU/1 -> ActivePowerModes/3(ActivePowerLimitOperatingParametersPU)
  ActivePowerSetPU/1 -> ActivePowerModes/4(ActivePowerSetPU)
  MaxDischargingPowerPU/1 -> ActivePowerModes/5(MaxDischargingPowerPU)
  DynamicVoltWattOperatingParametersPU/1 -> ActivePowerModes/17(DynamicVoltWattOperatingParametersPU)
  ActivePowerSmoothingOperatingParametersPU/1 -> ActivePowerModes/16(ActivePowerSmoothingOperatingParametersPU)
  FreqWattOperatingParametersPU/1 -> ActivePowerModes/15(FreqWattOperatingParametersPU)
  FreqMeasPU/1 -> ActivePowerModes/14(FreqPU)
  VoltWattOperatingParametersPU/1 -> ActivePowerModes/13(VoltWattOperatingParametersPU)
  VoltMeasPU/1 -> ActivePowerModes/12(VoltMeasPU)
  ActivePowerResponseOperatingParametersPU/1 -> ActivePowerModes/11(ActivePowerResponseOperatingParametersPU)
  ActivePowerMeasCtrlPointPU/1 -> ActivePowerModes/10(ActivePowerMeasCtrlPointPU)
  CrdChargeDischargeOperatingParametersPU/1 -> ActivePowerModes/9(CrdChargeDischargeOperatingParametersPU)
  MaxChargingPowerPU/1 -> ActivePowerModes/6(MaxChargingPowerPU)
  ActivePowerMeasPU/1 -> ActivePowerModes/7(ActivePowerMeasPU)
  SoCMeas/1 -> ActivePowerModes/8(SoCMeas)
  ReactivePowerControlMode/1 -> ReactivePowerModes/1(ReactivePowerControlMode)
  ReactivePowerSetPU/1 -> ReactivePowerModes/2(ReactivePowerSetPU)
  PowerFactorSet/1 -> ReactivePowerModes/3(PowerFactorSet)
  ActivePowerMeasPU1/1 -> ReactivePowerModes/4(ActivePowerMeasPU)
  VoltMeasPU1/1 -> ReactivePowerModes/5(VoltMeasPU)
  VoltVAROperatingParametersPU/1 -> ReactivePowerModes/6(VoltVAROperatingParametersPU)
  WattVAROperatingParametersPU/1 -> ReactivePowerModes/7(WattVAROperatingParametersPU)

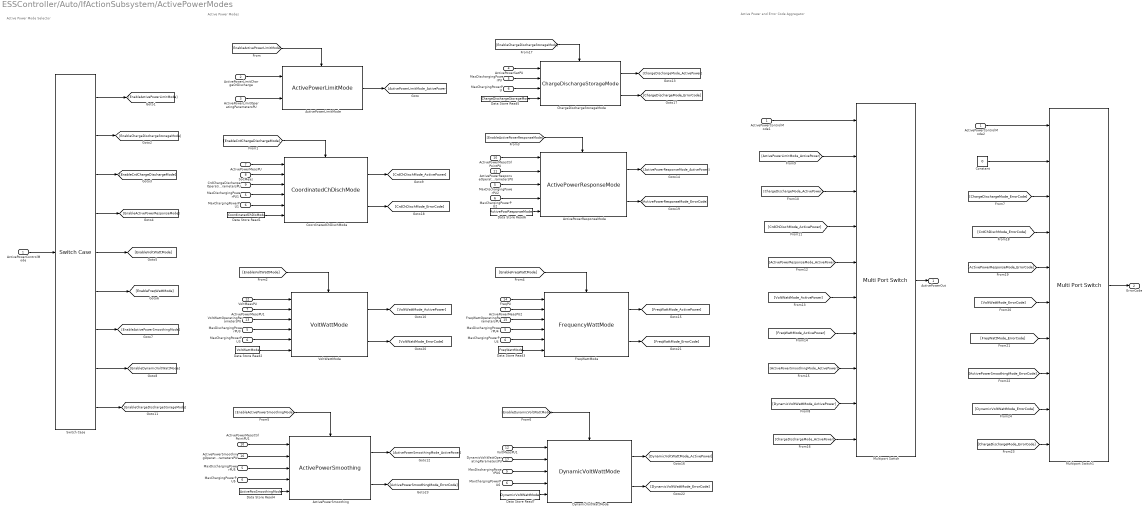
== system ESSController/Auto/IfActionSubsystem/ActivePowerModes ==
  note: Active Power and Error Code Aggregator
  note: Active Power Modes
  note: Active Power Mode Selector
  ActivePowerControlMode : Inport
  ActivePowerLimitChargeOrDischarge : Inport  Port=2
  ActivePowerLimitOperatingParametersPU : Inport  Port=3  OutDataTypeStr=Bus: ActivePowerLimitOperatingParametersPU
  ActivePowerSetPU : Inport  Port=4
  MaxDischargingPowerPU : Inport  Port=5
  MaxChargingPowerPU : Inport  Port=6
  ActivePowerMeasPU : Inport  Port=7
  SoCMeas : Inport  Port=8
  CrdChargeDischargeOperatingParametersPU : Inport  Port=9  OutDataTypeStr=Bus: CrdChargeDischargeOperatingParametersPU
  ActivePowerMeasCtrlPointPU : Inport  Port=10
  ActivePowerResponseOperatingParametersPU : Inport  Port=11  OutDataTypeStr=Bus: ActivePowerResponseOperatingParametersPU
  VoltMeasPU : Inport  Port=12
  VoltWattOperatingParametersPU : Inport  Port=13  OutDataTypeStr=Bus: VoltWattOperatingParametersPU
  FreqPU : Inport  Port=14
  FreqWattOperatingParametersPU : Inport  Port=15  OutDataTypeStr=Bus: FreqWattOperatingParametersPU
  ActivePowerSmoothingOperatingParametersPU : Inport  Port=16  OutDataTypeStr=Bus: ActivePowerSmoothingOperatingParametersPU
  DynamicVoltWattOperatingParametersPU : Inport  Port=17  OutDataTypeStr=Bus: DynamicVoltWattOperatingParametersPU
  ActivePowerControlMode1 : InportShadow
  ActivePowerControlMode2 : InportShadow
  ActivePowerLimitMode : ESSLibrary/ActivePowerLimitMode  SystemSampleTime=-1  Latency=0  AutoFrameSizeCalculation=off
  ActivePowerMeasCtrlPointPU1 : InportShadow  Port=10
  ActivePowerMeasPU1 : InportShadow  Port=7
  ActivePowerMeasPU2 : InportShadow  Port=7
  ActivePowerResponseMode : ESSLibrary/ActivePowerResponseMode  SystemSampleTime=-1  Latency=0  AutoFrameSizeCalculation=off
  ActivePowerSmoothing : ESSLibrary/ActivePowerSmoothing  SystemSampleTime=-1  Latency=0  AutoFrameSizeCalculation=off
  ChargeDischargeStorageMode : ESSLibrary/ChargeDischargeStorageMode  SystemSampleTime=-1  Latency=0  AutoFrameSizeCalculation=off
  Constant : Constant  Value=0  OutDataTypeStr=int32
  CoordinatedChDischMode : ESSLibrary/CoordinatedChDischMode  SystemSampleTime=-1  Latency=0  AutoFrameSizeCalculation=off
  Data Store Read1 : DataStoreRead  DataStoreName=CoordinatedChDisMode
  Data Store Read2 : DataStoreRead  DataStoreName=VoltWattMode
  Data Store Read3 : DataStoreRead  DataStoreName=FreqWattMode
  Data Store Read4 : DataStoreRead  DataStoreName=ActivePowSmoothingMode
  Data Store Read5 : DataStoreRead  DataStoreName=ChargeDischargeStorageMode
  Data Store Read6 : DataStoreRead  DataStoreName=ActivePowResponseMode
  Data Store Read7 : DataStoreRead  DataStoreName=DynamicVoltWattMode
  DynamicVoltWattMode : ESSLibrary/DynamicVoltWattMode  SystemSampleTime=-1  Latency=0  AutoFrameSizeCalculation=off
  FreqWattMode : ESSLibrary/FrequencyWattMode  SystemSampleTime=-1  Latency=0  AutoFrameSizeCalculation=off
  MaxChargingPowerPU{1..6} (6 alike) : InportShadow  Port=6
  MaxDischargingPowerPU{1..6} (6 alike) : InportShadow  Port=5
  Multiport Switch : MultiPortSwitch  Inputs=9
  Multiport Switch1 : MultiPortSwitch  Inputs=9
  Switch Case : SwitchCase  CaseConditions={1,2,3,4,5,6,7,8}
  VoltMeasPU1 : InportShadow  Port=12
  VoltWattMode : ESSLibrary/VoltWattMode  SystemSampleTime=-1  Latency=0  AutoFrameSizeCalculation=off
  ActivePowerOut : Outport
  ErrorCode : Outport  Port=2
  wires:
  ActivePowerControlMode/1 -> Switch Case/1
  Switch Case/6 -> [EnableFreqWattMode]
  Switch Case/5 -> [EnableVoltWattMode]
  Switch Case/4 -> [EnableActivePowerResponseMode]
  Switch Case/1 -> [EnableActivePowerLimitMode]
  Switch Case/3 -> [EnableCrdChargeDischargeMode]
  Switch Case/2 -> [EnableChargeDischargeStorageMode]
  Switch Case/8 -> [EnableDynamicVoltWattMode]
  Switch Case/9 -> [EnableChargeDischargeStorageMode]
  Switch Case/7 -> [EnableActivePowerSmoothingMode]
  ActivePowerLimitChargeOrDischarge/1 -> ActivePowerLimitMode/1
  ActivePowerLimitOperatingParametersPU/1 -> ActivePowerLimitMode/2
  ActivePowerSetPU/1 -> ChargeDischargeStorageMode/1
  MaxDischargingPowerPU/1 -> ChargeDischargeStorageMode/2
  MaxChargingPowerPU/1 -> ChargeDischargeStorageMode/3
  [EnableChargeDischargeStorageMode] -> ChargeDischargeStorageMode/Action
  Data Store Read5/1 -> ChargeDischargeStorageMode/4
  ActivePowerMeasPU/1 -> CoordinatedChDischMode/1
  SoCMeas/1 -> CoordinatedChDischMode/2
  CrdChargeDischargeOperatingParametersPU/1 -> CoordinatedChDischMode/3
  MaxDischargingPowerPU1/1 -> CoordinatedChDischMode/4
  MaxChargingPowerPU1/1 -> CoordinatedChDischMode/5
  Data Store Read1/1 -> CoordinatedChDischMode/6
  [EnableCrdChargeDischargeMode] -> CoordinatedChDischMode/Action
  [EnableActivePowerResponseMode] -> ActivePowerResponseMode/Action
  [EnableActivePowerLimitMode] -> ActivePowerLimitMode/Action
  ActivePowerMeasCtrlPointPU/1 -> ActivePowerResponseMode/1
  ActivePowerResponseOperatingParametersPU/1 -> ActivePowerResponseMode/2
  MaxDischargingPowerPU2/1 -> ActivePowerResponseMode/3
  MaxChargingPowerPU2/1 -> ActivePowerResponseMode/4
  Data Store Read6/1 -> ActivePowerResponseMode/5
  [EnableVoltWattMode] -> VoltWattMode/Action
  VoltMeasPU/1 -> VoltWattMode/1
  ActivePowerMeasPU1/1 -> VoltWattMode/2
  VoltWattOperatingParametersPU/1 -> VoltWattMode/3
  MaxDischargingPowerPU3/1 -> VoltWattMode/4
  MaxChargingPowerPU3/1 -> VoltWattMode/5
  Data Store Read2/1 -> VoltWattMode/6
  [EnableFreqWattMode] -> FreqWattMode/Action
  FreqPU/1 -> FreqWattMode/1
  ActivePowerMeasPU2/1 -> FreqWattMode/2
  FreqWattOperatingParametersPU/1 -> FreqWattMode/3
  MaxDischargingPowerPU4/1 -> FreqWattMode/4
  MaxChargingPowerPU4/1 -> FreqWattMode/5
  Data Store Read3/1 -> FreqWattMode/6
  [EnableActivePowerSmoothingMode] -> ActivePowerSmoothing/Action
  ActivePowerMeasCtrlPointPU1/1 -> ActivePowerSmoothing/1
  ActivePowerSmoothingOperatingParametersPU/1 -> ActivePowerSmoothing/2
  MaxDischargingPowerPU5/1 -> ActivePowerSmoothing/3
  MaxChargingPowerPU5/1 -> ActivePowerSmoothing/4
  Data Store Read4/1 -> ActivePowerSmoothing/5
  [EnableDynamicVoltWattMode] -> DynamicVoltWattMode/Action
  VoltMeasPU1/1 -> DynamicVoltWattMode/1
  DynamicVoltWattOperatingParametersPU/1 -> DynamicVoltWattMode/2
  MaxDischargingPowerPU6/1 -> DynamicVoltWattMode/3
  MaxChargingPowerPU6/1 -> DynamicVoltWattMode/4
  Data Store Read7/1 -> DynamicVoltWattMode/5
  ActivePowerLimitMode/1 -> [ActivePowerLimitMode_ActivePower]
  CoordinatedChDischMode/1 -> [CrdChDischMode_ActivePower]
  VoltWattMode/1 -> [VoltWattMode_ActivePower]
  ActivePowerSmoothing/1 -> [ActivePowerSmoothingMode_ActivePower]
  ChargeDischargeStorageMode/1 -> [ChargeDischargeMode_ActivePower]
  ActivePowerResponseMode/1 -> [ActivePowerResponseMode_ActivePower]
  FreqWattMode/1 -> [FreqWattMode_ActivePower]
  DynamicVoltWattMode/1 -> [DynamicVoltWattMode_ActivePower]
  [DynamicVoltWattMode_ActivePower] -> Multiport Switch/9
  [ActivePowerSmoothingMode_ActivePower] -> Multiport Switch/8
  ActivePowerControlMode1/1 -> Multiport Switch/1
  [FreqWattMode_ActivePower] -> Multiport Switch/7
  [ActivePowerResponseMode_ActivePower] -> Multiport Switch/5
  [VoltWattMode_ActivePower] -> Multiport Switch/6
  [ChargeDischargeMode_ActivePower] -> Multiport Switch/3
  [CrdChDischMode_ActivePower] -> Multiport Switch/4
  [ActivePowerLimitMode_ActivePower] -> Multiport Switch/2
  [ChargeDischargeMode_ActivePower] -> Multiport Switch/10
  Multiport Switch/1 -> ActivePowerOut/1
  ActivePowerControlMode2/1 -> Multiport Switch1/1
  ChargeDischargeStorageMode/2 -> [ChargeDischargeMode_ErrorCode]
  CoordinatedChDischMode/2 -> [CrdChDischMode_ErrorCode]
  ActivePowerResponseMode/2 -> [ActivePowerResponseMode_ErrorCode]
  VoltWattMode/2 -> [VoltWattMode_ErrorCode]
  FreqWattMode/2 -> [FreqWattMode_ErrorCode]
  DynamicVoltWattMode/2 -> [DynamicVoltWattMode_ErrorCode]
  ActivePowerSmoothing/2 -> [ActivePowerSmoothingMode_ErrorCode]
  [ActivePowerSmoothingMode_ErrorCode] -> Multiport Switch1/8
  [DynamicVoltWattMode_ErrorCode] -> Multiport Switch1/9
  [ActivePowerResponseMode_ErrorCode] -> Multiport Switch1/5
  [FreqWattMode_ErrorCode] -> Multiport Switch1/7
  [ChargeDischargeMode_ErrorCode] -> Multiport Switch1/10
  [VoltWattMode_ErrorCode] -> Multiport Switch1/6
  [CrdChDischMode_ErrorCode] -> Multiport Switch1/4
  [ChargeDischargeMode_ErrorCode] -> Multiport Switch1/3
  Constant/1 -> Multiport Switch1/2
  Multiport Switch1/1 -> ErrorCode/1

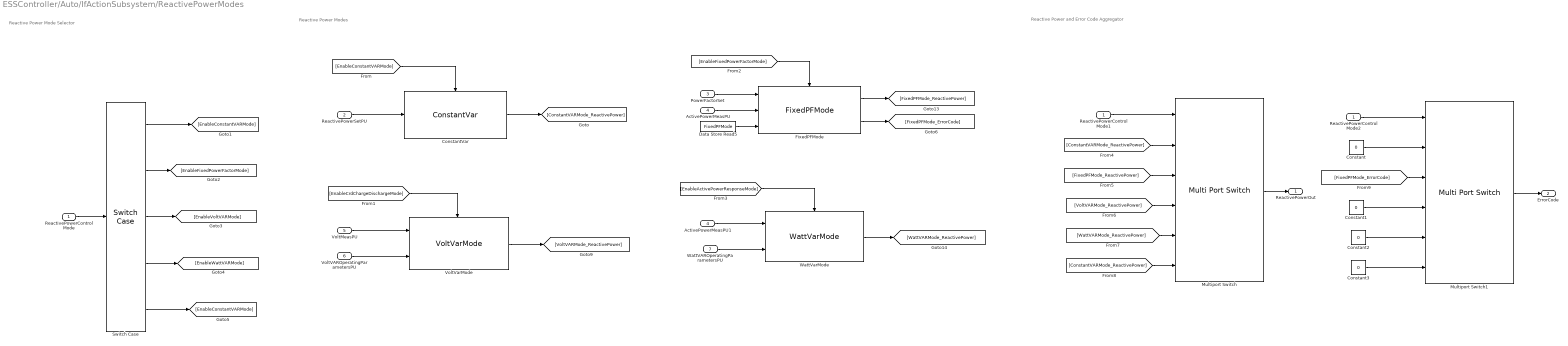
== system ESSController/Auto/IfActionSubsystem/ReactivePowerModes ==
  note: Reactive Power Mode Selector
  note: Reactive Power Modes
  note: Reactive Power and Error Code Aggregator
  ReactivePowerControlMode : Inport
  ReactivePowerSetPU : Inport  Port=2
  PowerFactorSet : Inport  Port=3
  ActivePowerMeasPU : Inport  Port=4
  VoltMeasPU : Inport  Port=5
  VoltVAROperatingParametersPU : Inport  Port=6  OutDataTypeStr=Bus: VoltVarOperatingParametersPU
  WattVAROperatingParametersPU : Inport  Port=7  OutDataTypeStr=Bus: WattVarOperatingParametersPU
  ActivePowerMeasPU1 : InportShadow  Port=4
  Constant{,1..3} (4 alike) : Constant  Value=0  OutDataTypeStr=int32
  ConstantVar : ESSLibrary/ConstantVar  SystemSampleTime=-1  Latency=0  AutoFrameSizeCalculation=off
  Data Store Read5 : DataStoreRead  DataStoreName=FixedPFMode
  FixedPFMode : ESSLibrary/FixedPFMode  SystemSampleTime=-1  Latency=0  AutoFrameSizeCalculation=off
  Multiport Switch : MultiPortSwitch  Inputs=5
  Multiport Switch1 : MultiPortSwitch  Inputs=5
  ReactivePowerControlMode1 : InportShadow
  ReactivePowerControlMode2 : InportShadow
  Switch Case : SwitchCase  CaseConditions={1,2,3,4}
  VoltVarMode : ESSLibrary/VoltVarMode  SystemSampleTime=-1  Latency=0  AutoFrameSizeCalculation=off
  WattVarMode : ESSLibrary/WattVarMode  SystemSampleTime=-1  Latency=0  AutoFrameSizeCalculation=off
  ReactivePowerOut : Outport
  ErrorCode : Outport  Port=2
  wires:
  Multiport Switch/1 -> ReactivePowerOut/1
  Multiport Switch1/1 -> ErrorCode/1
  [EnableConstantVARMode] -> ConstantVar/Action
  ConstantVar/1 -> [ConstantVARMode_ReactivePower]
  [EnableActivePowerResponseMode] -> WattVarMode/Action
  ? -> ?
  Switch Case/1 -> [EnableConstantVARMode]
  Switch Case/3 -> [EnableVoltVARMode]
  ReactivePowerControlMode1/1 -> Multiport Switch/1
  [EnableCrdChargeDischargeMode] -> VoltVarMode/Action
  ReactivePowerControlMode/1 -> Switch Case/1
  [EnableFixedPowerFactorMode] -> FixedPFMode/Action
  Switch Case/2 -> [EnableFixedPowerFactorMode]
  WattVarMode/1 -> [WattVARMode_ReactivePower]
  Switch Case/4 -> [EnableWattVARMode]
  Switch Case/5 -> [EnableConstantVARMode]
  ReactivePowerSetPU/1 -> ConstantVar/1
  FixedPFMode/1 -> [FixedPFMode_ReactivePower]
  FixedPFMode/2 -> [FixedPFMode_ErrorCode]
  PowerFactorSet/1 -> FixedPFMode/1
  ActivePowerMeasPU/1 -> FixedPFMode/2
  Data Store Read5/1 -> FixedPFMode/3
  VoltMeasPU/1 -> VoltVarMode/1
  VoltVAROperatingParametersPU/1 -> VoltVarMode/2
  VoltVarMode/1 -> [VoltVARMode_ReactivePower]
  ActivePowerMeasPU1/1 -> WattVarMode/1
  WattVAROperatingParametersPU/1 -> WattVarMode/2
  [ConstantVARMode_ReactivePower] -> Multiport Switch/2
  [FixedPFMode_ReactivePower] -> Multiport Switch/3
  [VoltVARMode_ReactivePower] -> Multiport Switch/4
  [WattVARMode_ReactivePower] -> Multiport Switch/5
  [ConstantVARMode_ReactivePower] -> Multiport Switch/6
  ReactivePowerControlMode2/1 -> Multiport Switch1/1
  [FixedPFMode_ErrorCode] -> Multiport Switch1/3
  Constant/1 -> Multiport Switch1/2
  Constant1/1 -> Multiport Switch1/4
  Constant2/1 -> Multiport Switch1/5
  Constant3/1 -> Multiport Switch1/6
